simulink model "hardware_velo_control"  (R2020b)
settings: Solver=ode1  StartTime=0.0  StopTime=30  FixedStep=0.01  RelTol=1e-3  EnableMultiTasking=on
libraries: arduinolib x2, pid_lib x1
settings Model: SILPILModeSetting=veronly  ExtModeTrigDuration=2  Creator=ONLY-GOD  LastModifiedBy=ONLY-GOD
settings OptimizationCC: EnhancedBackFolding=on  PassReuseOutputArgsAs=Individual arguments  ZeroExternalMemoryAtStartup=off  ZeroInternalMemoryAtStartup=off  MaxStackSize=64  OptimizeBlockOrder=speed  DifferentSizesBufferReuse=on  EfficientTunableParamExpr=on
settings DebuggingCC: ParameterTunabilityLossMsg=error
settings HardwareCC: ProdBitPerPointer=32  ProdBitPerSizeT=32  ProdBitPerPtrDiffT=32  ProdLargestAtomicInteger=Long  ProdLargestAtomicFloat=Double  ProdWordSize=32  ProdHWDeviceType=ARM Compatible->ARM Cortex
settings SFSimCC: MATLABDynamicMemAlloc=off
settings RTWCC: Description=Embedded Coder  SystemTargetFile=ert.tlc  HardwareBoard=Arduino Due  TLCOptions="-aInlineSetEventsForThisBaseRateFcn=TLC_FALSE -aSuppressMultiTaskScheduler=TLC_FALSE   -aRateBasedStepFcn=1"  TemplateMakefile=ert_default_tmf  Toolchain=Arduino ARM  BuildConfiguration=Faster Runs
settings CodeAppCC: ForceParamTrailComments=on  IgnoreCustomStorageClasses=off  OperatorAnnotations=on  SimulinkDataObjDesc=on  SFDataObjDesc=on  InsertBlockDesc=on
settings ERTTargetCC: SupportContinuousTime=on  SupportVariableSizeSignals=on  ExtModeTransport=3  ExtModeStaticAllocSize=24576  ExtModeMexFile=ext_xcp  ExtModeIntrfLevel=Level2 - Open

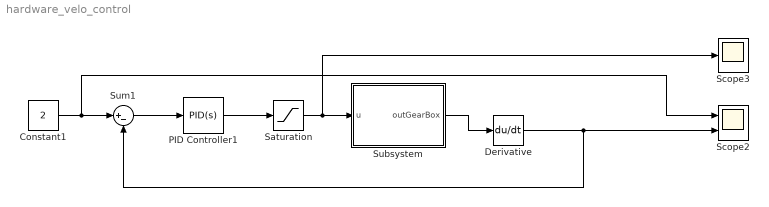
== system hardware_velo_control ==
  Constant1 : Constant  Value=2
  Derivative : Derivative
  PID Controller1 : pid_lib/PID Controller  Controller=PID  Form=Parallel  TimeDomain=Continuous-time  UseExternalTs=off  SampleTime=-1  IntegratorMethod=Forward Euler  FilterMethod=Forward Euler  ControllerParametersSource=internal  P=7  I=5  D=0.4  UseFilter=on  N=0  TunerSelectOption=Transfer Function Based (PID Tuner App)  InitialConditionSource=internal  InitialConditionForIntegrator=0  InitialConditionForFilter=0  DifferentiatorICPrevScaledInput=0  ExternalReset=none  TrackingMode=off  Kt=1  LimitOutput=off  SatLimitsSource=internal  UpperSaturationLimit=inf  LowerSaturationLimit=-inf  LinearizeAsGain=on  AntiWindupMode=none  Kb=1  POutMin=[]  POutMax=[]  IOutMin=[]  IOutMax=[]  DOutMin=[]  DOutMax=[]  NOutMin=[]  NOutMax=[]  SumOutMin=[]  SumOutMax=[]  SaturationOutMin=[]  SaturationOutMax=[]  PParamMin=[]  PParamMax=[]  IParamMin=[]  IParamMax=[]  DParamMin=[]  DParamMax=[]  NParamMin=[]  NParamMax=[]  KbParamMin=[]  KbParamMax=[]  KtParamMin=[]  KtParamMax=[]  KbOutMin=[]  KbOutMax=[]  KtOutMin=[]  KtOutMax=[]  IntegratorOutMin=[]  IntegratorOutMax=[]  FilterOutMin=[]  FilterOutMax=[]  SumI1OutMin=[]  SumI1OutMax=[]  SumI2OutMin=[]  SumI2OutMax=[]  SumI3OutMin=[]  SumI3OutMax=[]  SumI4OutMin=[]  SumI4OutMax=[]  SumDOutMin=[]  SumDOutMax=[]  DifferentiatorOutMin=[]  DifferentiatorOutMax=[]  FilterDiffOutCoefMin=[]  FilterDiffOutCoefMax=[]  ReciprocalOutMin=[]  ReciprocalOutMax=[]  SumDenOutMin=[]  SumDenOutMax=[]  SumNumOutMin=[]  SumNumOutMax=[]  DivideOutMin=[]  DivideOutMax=[]  UdiffTsProdOutMin=[]  UdiffTsProdOutMax=[]  NTsProdOutMin=[]  NTsProdOutMax=[]  UintegralTsProdOutMin=[]  UintegralTsProdOutMax=[]  UngainTsProdOutMin=[]  UngainTsProdOutMax=[]  IntegratorContinuousStateAttributes=''  IntegratorStateMustResolveToSignalObject=off  IntegratorRTWStateStorageClass=Auto  FilterContinuousStateAttributes=''  FilterStateMustResolveToSignalObject=off  FilterRTWStateStorageClass=Auto  ParallelPVariant=InternalParameters  IdealPVariant=Disabled  IVariant=InternalParameters  DVariant=InternalParameters  IntegratorVariant=Continuous  SatVariant=Disabled  AWVariant=Passthrough  PCopyVariant=Disabled  TRVariant=Disabled  FdbkBlocksVariant=Forward  IdealPFdbkVariant=Disabled  SatFdbkVariant=Disabled  DerivativeFilterVariant=ContFilter  NVariant=InternalParameters  NCopyVariant=Disabled  FilterICVariant=InternalICsFilter  IntegratorICVariant=InternalICs  ExternalResetVariant=Disabled  TRSumVariant=Passthrough  SumFdbkVariant=Disabled  SumVariant=Sum_PID  TsampFilterVariant=InternalTs  TsampNgainVariant=Passthrough  TsampIntegralVariant=Passthrough  ExternalSaturationOutDataTypeStr=Inherit: Same as second input
  Saturation : Saturate  UpperLimit=24  LowerLimit=-24
  Scope2 : Scope  NumInputPorts=2
  Scope3 : Scope
  Subsystem : Subsystem
  Sum1 : Sum  Inputs=|+-
  wires:
  Constant1/1 -> Sum1/1, Scope2/1
  Sum1/1 -> PID Controller1/1
  Derivative/1 -> Scope2/2, Sum1/2
  PID Controller1/1 -> Saturation/1
  Saturation/1 -> Subsystem/1(u), Scope3/1
  Subsystem/1(outGearBox) -> Derivative/1

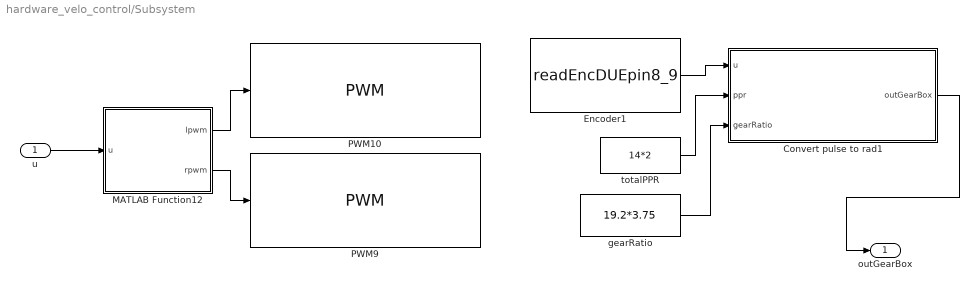
== system hardware_velo_control/Subsystem ==
  u : Inport
  Convert pulse to rad1 : MATLAB Function  TreatAsAtomicUnit=on
  Encoder1 : S-Function  InitFcn=try, set_param(gcb,'FunctionName','readEncDUEpin8_9'), end  FunctionName=readEncDUEpin8_9  SFunctionModules=readEncDUEpin8_9_wrapper  SFunctionDeploymentMode=off  EnableBusSupport=off  mask(S-Function Builder){}
      mask help: Simulink:masks:SFunctionBuilder_MD
      mask init:
      | val = [[.9  0.75 0.75 1 1 .9 .9 1]',[1 1 0.75 0.75 .9 .9 1 .9]'];try , sys = get_param(gcb,'SfunBuilderFcnName');if isempty(sys), sys = get_param(gcb,'FunctionName'); end,catch, sys = get_param(gcb,'FunctionName'); end
      settings: CopyFcn=set_param(gcbh,'LinkStatus','none')  PreSaveFcn=try, set_param(gcb,'FunctionName','readEncDUEpin8_9'), end  OpenFcn=sfunctionwizard(gcbh)
      mask Display: plot(val(:,1),val(:,2)),disp(sys),port_label('output',1,'count')
  MATLAB Function12 : MATLAB Function  TreatAsAtomicUnit=on
  PWM10 : arduinolib/PWM  pinNumber=7  frequencyType=Default  desiredFrequency=490.2  achievableFrequency=490.2
  PWM9 : arduinolib/PWM  pinNumber=6  frequencyType=Default  desiredFrequency=490.2  achievableFrequency=490.2
  gearRatio : Constant  Value=19.2*3.75
  totalPPR : Constant  Value=14*2
  outGearBox : Outport
  wires:
  Encoder1/1 -> Convert pulse to rad1/1(u)
  MATLAB Function12/1(lpwm) -> PWM10/1
  totalPPR/1 -> Convert pulse to rad1/2(ppr)
  MATLAB Function12/2(rpwm) -> PWM9/1
  gearRatio/1 -> Convert pulse to rad1/3(gearRatio)
  u/1 -> MATLAB Function12/1(u)
  Convert pulse to rad1/1(outGearBox) -> outGearBox/1

== matlab function hardware_velo_control/Subsystem/MATLAB Function12 ==
  data: u input; lpwm output; rpwm output
function [lpwm,rpwm] = fcn(u)

Vmax = 22.9;
pwm = u*254/Vmax;
if pwm > 0
    lpwm = pwm;
    rpwm = 0;
elseif pwm < 0
    lpwm = 0;
    rpwm = abs(pwm);
else
    lpwm = 0;
    rpwm = 0;
end

== matlab function hardware_velo_control/Subsystem/Convert pulse to rad1 ==
  settings: updateMethod=DISCRETE
  data: u input; ppr input; gearRatio input; outGearBox output
function outGearBox = fcn(u,ppr,gearRatio)

persistent counter_num over_flag
if(isempty(counter_num)), counter_num = 0;end
if(isempty(over_flag)), over_flag = 0;end
pulse2radian = 2*pi/ppr; % 1 pulse = ?? radian

if(double(u) - counter_num > 40000), over_flag = over_flag-1;
elseif(double(u) - counter_num < -40000), over_flag = over_flag+1;
end

inGearBox = (double(u)+over_flag*(2^32 -1))*pulse2radian; 
outGearBox = inGearBox/gearRatio;
counter_num = double(u) ;
